simulink model "on_off_control"  (R2017b)
settings: Solver=VariableStepAuto  StartTime=0.0  StopTime=1  RelTol=1e-3
settings Model: Creator=Damla  LastModifiedBy=dagac
settings OptimizationCC: BlockReduction=off  DefaultParameterBehavior=Inlined  BufferReuse=off

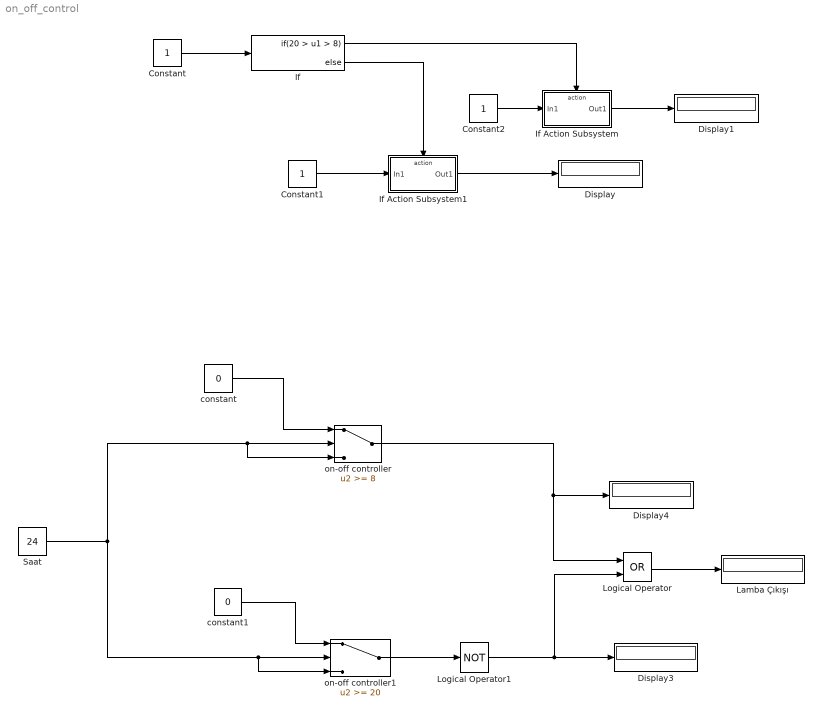
== system on_off_control ==
  Constant : Constant
  Constant1 : Constant
  Constant2 : Constant
  Display{,1,3..4} (4 alike) : Display
  If : If  IfExpression=20 > u1 > 8
  If Action Subsystem : Subsystem  TreatAsAtomicUnit=on
  If Action Subsystem1 : Subsystem  TreatAsAtomicUnit=on
  Lamba Çıkışı : Display
  Logical Operator : Logic  Operator=OR  AllPortsSameDT=off  OutDataTypeStr=boolean
  Logical Operator1 : Logic  Operator=NOT  Inputs=1  AllPortsSameDT=off  OutDataTypeStr=boolean
  Saat : Constant  Value=24
  constant : Constant  Value=0
  constant1 : Constant  Value=0
  on-off controller : Switch  Threshold=8
  on-off controller1 : Switch  Threshold=20
  wires:
  If/1 -> If Action Subsystem/Action
  Constant/1 -> If/1
  If/2 -> If Action Subsystem1/Action
  Constant1/1 -> If Action Subsystem1/1(In1)
  If Action Subsystem1/1(Out1) -> Display/1
  If Action Subsystem/1(Out1) -> Display1/1
  Constant2/1 -> If Action Subsystem/1(In1)
  constant/1 -> on-off controller/1
  on-off controller/1 -> Logical Operator/1, Display4/1
  Saat/1 -> on-off controller/3, on-off controller/2, on-off controller1/3, on-off controller1/2
  constant1/1 -> on-off controller1/1
  on-off controller1/1 -> Logical Operator1/1
  Logical Operator/1 -> Lamba Çıkışı/1
  Logical Operator1/1 -> Display3/1, Logical Operator/2

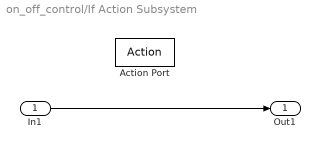
== system on_off_control/If Action Subsystem ==
  In1 : Inport
  Action Port : ActionPort  ActionType=then
  Out1 : Outport
  wires:
  In1/1 -> Out1/1

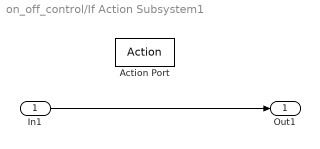
== system on_off_control/If Action Subsystem1 ==
  In1 : Inport
  Action Port : ActionPort  ActionType=else
  Out1 : Outport
  wires:
  In1/1 -> Out1/1
